simulink model "M1_P3_A_2"  (R2023a)
settings: Solver=VariableStepAuto  StartTime=0.0  StopTime=2.5  RelTol=1e-3
undefined symbols (not defined in the file): f_eff, J_eff, Kb, Ktn, L, R
settings Model: Creator=azzam  LastModifiedBy=azzam

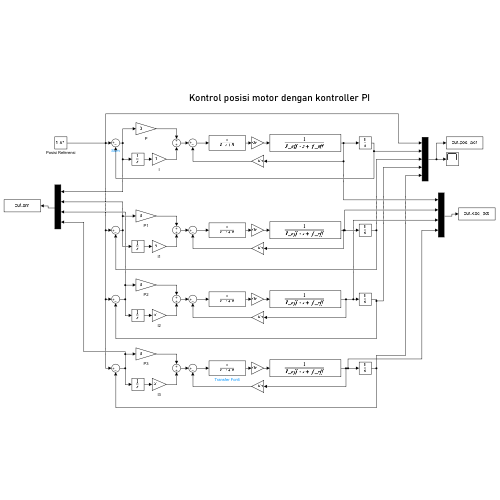
[thumbnail: Simulink's stored preview of the top-level diagram]
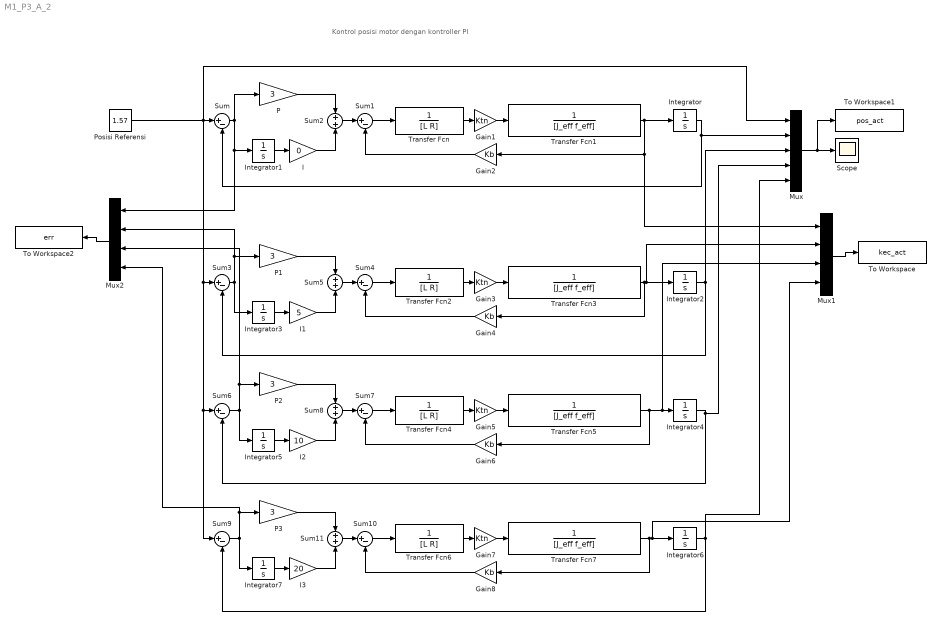
== system M1_P3_A_2 ==
  note: Kontrol posisi motor dengan kontroller PI
  Gain{1,3,5,7} (4 alike) : Gain  Gain=Ktn
  Gain{2,4,6,8} (4 alike) : Gain  Gain=Kb
  I : Gain  Gain=0
  I1 : Gain  Gain=5
  I2 : Gain  Gain=10
  I3 : Gain  Gain=20
  Integrator{,1..7} (8 alike) : Integrator
  Mux : Mux  Inputs=5
  Mux1 : Mux
  Mux2 : Mux
  P{,1..3} (4 alike) : Gain  Gain=3
  Posisi Referensi : Constant  Value=1.57
  Scope : Scope
  Sum{,1,3..4,6..7,9..10} (8 alike) : Sum  Inputs=|+-
  Sum{2,5,8,11} (4 alike) : Sum
  To Workspace : ToWorkspace  VariableName=kec_act  SaveFormat=Timeseries  SampleTime=-1
  To Workspace1 : ToWorkspace  VariableName=pos_act  SaveFormat=Timeseries  SampleTime=-1
  To Workspace2 : ToWorkspace  VariableName=err  SaveFormat=Timeseries  SampleTime=-1
  Transfer Fcn{,2,4,6} (4 alike) : TransferFcn  Denominator=[L R]
  Transfer Fcn{1,3,5,7} (4 alike) : TransferFcn  Denominator=[J_eff f_eff]
  wires:
  Mux1/1 -> To Workspace/1
  Integrator/1 -> Sum/2, Mux/2
  Transfer Fcn1/1 -> Mux1/1, Gain2/1, Integrator/1
  Posisi Referensi/1 -> Sum9/1, Sum6/1, Sum3/1, Mux/1, Sum/1
  Transfer Fcn/1 -> Gain1/1
  Sum/1 -> Integrator1/1, Mux2/1, P/1
  Gain2/1 -> Sum1/2
  Gain1/1 -> Transfer Fcn1/1
  Sum1/1 -> Transfer Fcn/1
  Mux/1 -> To Workspace1/1, Scope/1
  Mux2/1 -> To Workspace2/1
  Sum2/1 -> Sum1/1
  P/1 -> Sum2/1
  I/1 -> Sum2/2
  Integrator1/1 -> I/1
  I1/1 -> Sum5/2
  P1/1 -> Sum5/1
  Sum3/1 -> Integrator3/1, Mux2/2, P1/1
  Sum4/1 -> Transfer Fcn2/1
  Gain4/1 -> Sum4/2
  Transfer Fcn2/1 -> Gain3/1
  Transfer Fcn3/1 -> Gain4/1, Mux1/2, Integrator2/1
  Integrator3/1 -> I1/1
  Gain3/1 -> Transfer Fcn3/1
  Sum5/1 -> Sum4/1
  Integrator2/1 -> Sum3/2, Mux/3
  Gain5/1 -> Transfer Fcn5/1
  Gain6/1 -> Sum7/2
  Integrator4/1 -> Mux/4, Sum6/2
  Integrator5/1 -> I2/1
  Transfer Fcn4/1 -> Gain5/1
  Sum7/1 -> Transfer Fcn4/1
  Sum8/1 -> Sum7/1
  Sum6/1 -> Integrator5/1, Mux2/3, P2/1
  Transfer Fcn5/1 -> Gain6/1, Mux1/3, Integrator4/1
  I2/1 -> Sum8/2
  P2/1 -> Sum8/1
  Gain7/1 -> Transfer Fcn7/1
  Gain8/1 -> Sum10/2
  Integrator6/1 -> Sum9/2, Mux/5
  Integrator7/1 -> I3/1
  Transfer Fcn6/1 -> Gain7/1
  Sum10/1 -> Transfer Fcn6/1
  Sum11/1 -> Sum10/1
  Sum9/1 -> Integrator7/1, Mux2/4, P3/1
  Transfer Fcn7/1 -> Gain8/1, Mux1/4, Integrator6/1
  I3/1 -> Sum11/2
  P3/1 -> Sum11/1
